simulink subsystem "Write_ULOG_Data_Fixed_Wing"  (R2025a)
settings: Solver=VariableStepAuto  StartTime=0.0  StopTime=10.0  RelTol=1e-3
libraries: px4Utilslib x1
settings Model: Creator=gurt1  LastModifiedBy=17036
settings RTWCC: GPUComputeCapability=3.5

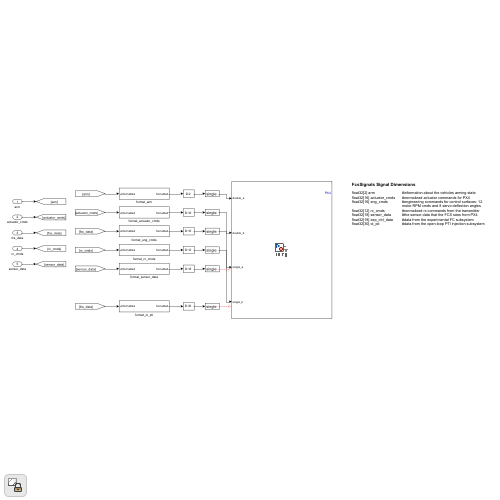
[thumbnail: Simulink's stored preview of the top-level diagram]
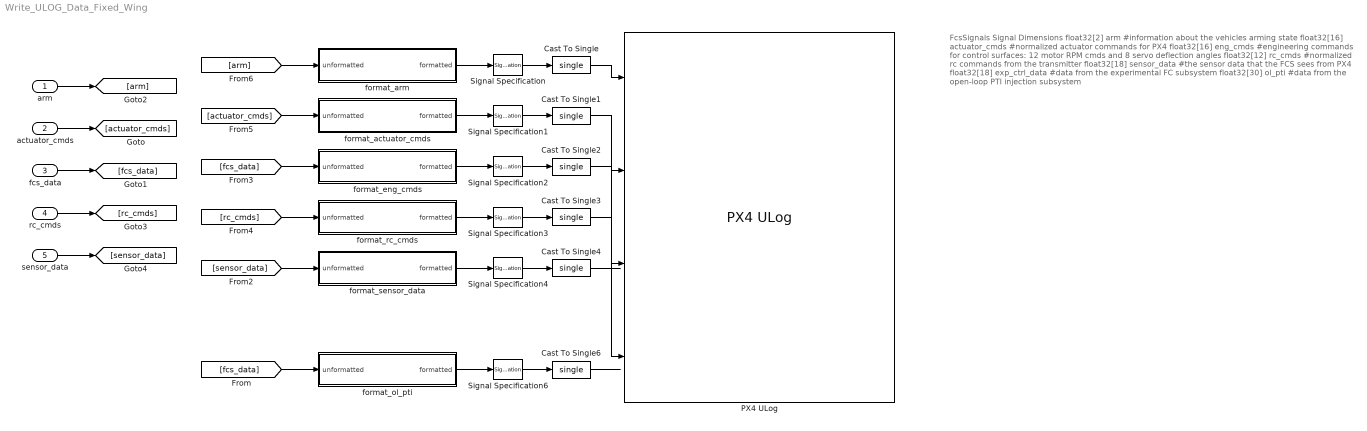
== system Write_ULOG_Data_Fixed_Wing ==
  note: FcsSignals Signal Dimensions
      |
      | float32[2] arm #information about the vehicles arming state
      | float32[16] actuator_cmds #normalized actuator commands for PX4
      | float32[16] eng_cmds #engineering commands for control surfaces: 12 motor RPM cmds and 8 servo deflection angles
      | float32[12] rc_cmds #normalized rc commands from the transmitter
      | float32[18] sensor_data #the sensor data that the FCS sees from PX4
      | float32[18] exp_ctrl_data #data from the experimental FC subsystem
      | float32[30] ol_pti #data from the open-loop PTI injection subsystem
  arm : Inport
  actuator_cmds : Inport  Port=2
  fcs_data : Inport  Port=3
  rc_cmds : Inport  Port=4
  sensor_data : Inport  Port=5
  Cast To Single{,1..4,6} (6 alike) : DataTypeConversion  OutDataTypeStr=single  SaturateOnIntegerOverflow=off  RndMeth=Floor
  PX4 ULog : px4Utilslib/PX4 ULog  uORBTopic=FcsSignals
  Signal Specification : SignalSpecification  Dimensions=2
  Signal Specification1 : SignalSpecification  Dimensions=16
  Signal Specification2 : SignalSpecification  Dimensions=16
  Signal Specification3 : SignalSpecification  Dimensions=12
  Signal Specification4 : SignalSpecification  Dimensions=18
  Signal Specification6 : SignalSpecification  Dimensions=30
  format_actuator_cmds : Subsystem
  format_arm : Subsystem
  format_eng_cmds : Subsystem
  format_ol_pti : Subsystem
  format_rc_cmds : Subsystem
  format_sensor_data : Subsystem
  wires:
  actuator_cmds/1 -> [actuator_cmds]
  arm/1 -> [arm]
  fcs_data/1 -> [fcs_data]
  sensor_data/1 -> [sensor_data]
  rc_cmds/1 -> [rc_cmds]
  [fcs_data] -> format_ol_pti/1(unformatted)
  [sensor_data] -> format_sensor_data/1(unformatted)
  [fcs_data] -> format_eng_cmds/1(unformatted)
  format_eng_cmds/1(formatted) -> Signal Specification2/1
  format_rc_cmds/1(formatted) -> Signal Specification3/1
  format_sensor_data/1(formatted) -> Signal Specification4/1
  [rc_cmds] -> format_rc_cmds/1(unformatted)
  format_actuator_cmds/1(formatted) -> Signal Specification1/1
  format_arm/1(formatted) -> Signal Specification/1
  [actuator_cmds] -> format_actuator_cmds/1(unformatted)
  [arm] -> format_arm/1(unformatted)
  format_ol_pti/1(formatted) -> Signal Specification6/1
  Signal Specification/1 -> Cast To Single/1
  Signal Specification1/1 -> Cast To Single1/1
  Signal Specification2/1 -> Cast To Single2/1
  Signal Specification3/1 -> Cast To Single3/1
  Signal Specification4/1 -> Cast To Single4/1
  Signal Specification6/1 -> Cast To Single6/1
  Cast To Single/1 -> PX4 ULog/1
  Cast To Single1/1 -> PX4 ULog/2
  Cast To Single2/1 -> PX4 ULog/3
  Cast To Single3/1 -> PX4 ULog/4
  Cast To Single4/1 -> ?
  Cast To Single6/1 -> ?

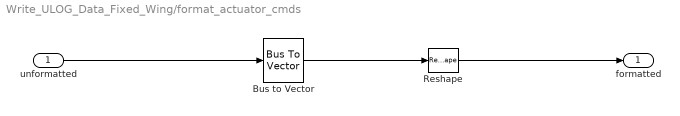
== system Write_ULOG_Data_Fixed_Wing/format_actuator_cmds ==
  unformatted : Inport
  Bus to Vector : BusToVector
  Reshape : Reshape
  formatted : Outport
  wires:
  Bus to Vector/1 -> Reshape/1
  Reshape/1 -> formatted/1
  unformatted/1 -> Bus to Vector/1

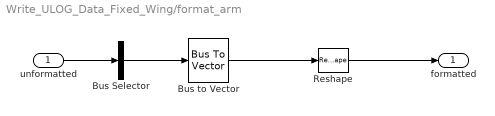
== system Write_ULOG_Data_Fixed_Wing/format_arm ==
  unformatted : Inport
  Bus Selector : BusSelector  OutputSignals=arm,dt_arm  OutputAsBus=on
  Bus to Vector : BusToVector
  Reshape : Reshape
  formatted : Outport
  wires:
  Bus to Vector/1 -> Reshape/1
  unformatted/1 -> Bus Selector/1
  Reshape/1 -> formatted/1
  Bus Selector/1 -> Bus to Vector/1

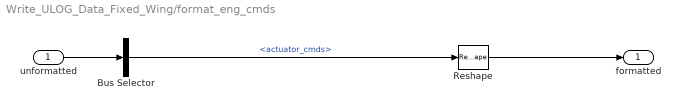
== system Write_ULOG_Data_Fixed_Wing/format_eng_cmds ==
  unformatted : Inport
  Bus Selector : BusSelector  OutputSignals=actuator_cmds
  Reshape : Reshape
  formatted : Outport
  wires:
  unformatted/1 -> Bus Selector/1
  Bus Selector/1 -> Reshape/1  "<actuator_cmds>"
  Reshape/1 -> formatted/1

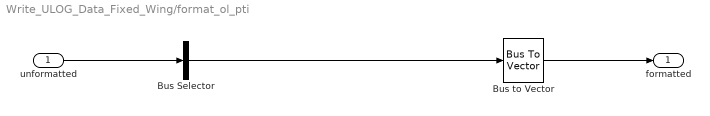
== system Write_ULOG_Data_Fixed_Wing/format_ol_pti ==
  unformatted : Inport
  Bus Selector : BusSelector  OutputSignals=OL_PTI  OutputAsBus=on
  Bus to Vector : BusToVector
  formatted : Outport
  wires:
  unformatted/1 -> Bus Selector/1
  Bus to Vector/1 -> formatted/1
  Bus Selector/1 -> Bus to Vector/1

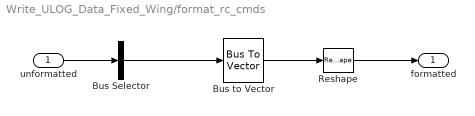
== system Write_ULOG_Data_Fixed_Wing/format_rc_cmds ==
  unformatted : Inport
  Bus Selector : BusSelector  OutputSignals=sticks,switches  OutputAsBus=on
  Bus to Vector : BusToVector
  Reshape : Reshape
  formatted : Outport
  wires:
  Reshape/1 -> formatted/1
  Bus Selector/1 -> Bus to Vector/1
  Bus to Vector/1 -> Reshape/1
  unformatted/1 -> Bus Selector/1

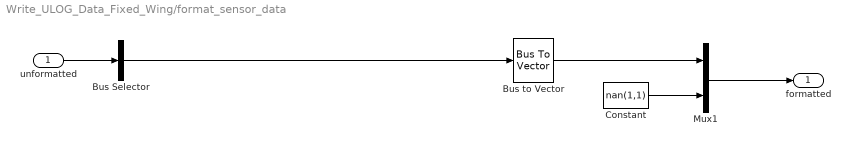
== system Write_ULOG_Data_Fixed_Wing/format_sensor_data ==
  unformatted : Inport
  Bus Selector : BusSelector  OutputSignals=att_rad,ang_rps,pos_ned_m,vel_ned_mps,alt_m,vt_kts,rho_kgmp3,flags  OutputAsBus=on
  Bus to Vector : BusToVector
  Constant : Constant  Value=nan(1,1)
  Mux1 : Mux  Inputs=2
  formatted : Outport
  wires:
  Mux1/1 -> formatted/1
  unformatted/1 -> Bus Selector/1
  Constant/1 -> Mux1/2
  Bus Selector/1 -> Bus to Vector/1
  Bus to Vector/1 -> Mux1/1
